simulink model "FowardDynamics_CDPR_20220518"  (R2020a)
settings: Solver=VariableStepAuto  StartTime=0.0  StopTime=12  FixedStep=0.01  RelTol=1e-3
undefined symbols (not defined in the file or in its folder): sigbuilder_block, X, Y, Z
libraries: sm_lib x197, nesl_utility x56, sm_cable_robot_lib x44, simulink x1
(part 2 of 8)

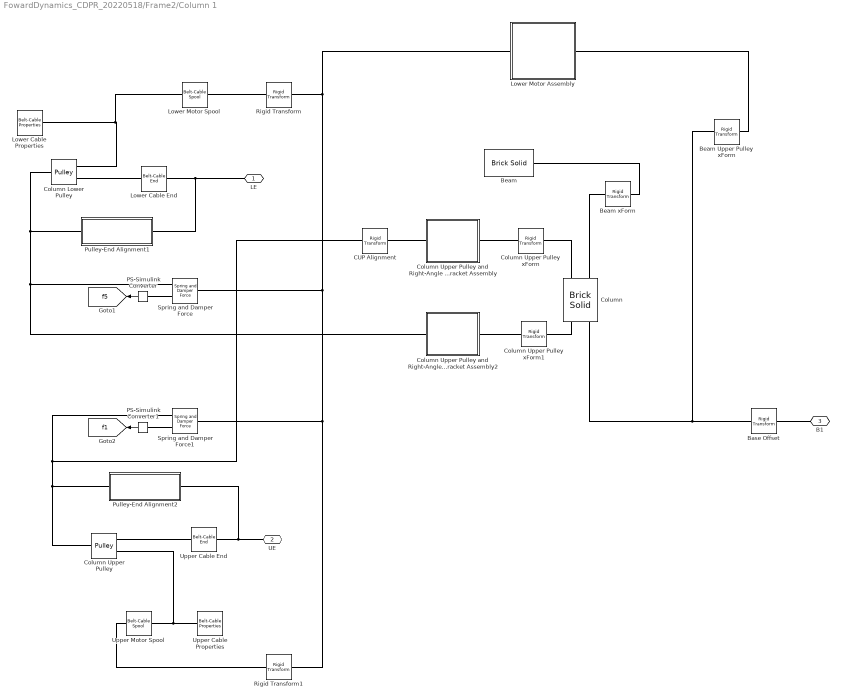
== system FowardDynamics_CDPR_20220518/Frame2/Column 1 ==
  Base Offset : sm_lib/Frames and Transforms/Rigid Transform  TranslationMethod=StandardAxis  TranslationStandardOffset=0  TranslationLengthUnit=m  TranslationStandardAxis=+X  TranslationCartesianOffset=[0 0 0]  TranslationROffset=0  TranslationROffsetUnits=m  TranslationZOffset=0  TranslationZOffsetUnits=m  TranslationThetaOffset=0  TranslationThetaOffsetUnits=deg  RotationMethod=None  RotationAngleUnits=deg  RotationStandardAxis=+Z  RotationAngle=0.0  RotationArbitraryAxis=[0 0 1]  FollAlignAxisA=+X  BaseAlignAxisA=+Y  FollAlignAxisB=+Y  BaseAlignAxisB=+Z  RotationSequenceAxes=FollowerAxes  RotationSequence=XYX  RotationSequenceAngles=[0 0 0]  RotationSequenceAnglesUnits=deg  RotationMatrix=[1 0 0; 0 1 0; 0 0 1]
  Beam : sm_lib/Body Elements/Brick Solid  GraphicAmbientColor=[0.15 0.15 0.15 1.0]  BasedOnType=Density  BrickDimensions=[0.1 2.1 0.1]  BrickDimensionUnits=m  CenterOfMass=[0 0 0]  CenterOfMassUnits=m  GraphicDiffuseColor=[0.4 0.4 0.4]  Density=7500  DensityUnits=kg/m^3  DoExposeReferenceFrame=off  GraphicEmissiveColor=[0.0 0.0 0.0 1.0]  ExportEntireGeometry=off  SerializedFrames=<Frames><Frame><Id>Frame3</Id><Value><Name>L</Name><Origin><Source>GeometricFeature</Source><FeatureName>-y surface</FeatureName></Origin><PrimaryAxis><DefinedDirection>+Z</DefinedDirection><Source>ReferenceFrame</Source><SourceDirection>+Z</SourceDirection><FeatureName></FeatureName></PrimaryAxis><SecondaryAxis><DefinedDirection>+X</DefinedDirection><Source>ReferenceFrame</Source><SourceDirection>+X</SourceDirection><FeatureName></FeatureName></SecondaryAxis></Value></Frame></Frames>  MarkerShape=Sphere  MarkerSize=10  GraphicType=FromGeometry  InertiaType=CalculateFromGeometry  Mass=1  MassUnits=kg  MomentsOfInertia=[1 1 1]  MomentsOfInertiaUnits=kg*m^2  GraphicOpacity=1.0  ProductsOfInertia=[0 0 0]  ProductsOfInertiaUnits=kg*m^2  GraphicShininess=75  GraphicSpecularColor=[0.5 0.5 0.5 1.0]  GraphicVisPropType=SimpleVisualProperties
  Beam Upper Pulley xForm : sm_lib/Frames and Transforms/Rigid Transform  TranslationMethod=Cartesian  TranslationStandardOffset=0.2  TranslationLengthUnit=m  TranslationStandardAxis=+X  TranslationCartesianOffset=[0.025 0.2 0]  TranslationROffset=0  TranslationROffsetUnits=m  TranslationZOffset=0  TranslationZOffsetUnits=m  TranslationThetaOffset=0  TranslationThetaOffsetUnits=deg  RotationMethod=RotationSequence  RotationAngleUnits=deg  RotationStandardAxis=+Y  RotationAngle=45  RotationArbitraryAxis=[0 0 1]  FollAlignAxisA=+X  BaseAlignAxisA=+Z  FollAlignAxisB=+Y  BaseAlignAxisB=-X  RotationSequenceAxes=FollowerAxes  RotationSequence=XYZ  RotationSequenceAngles=[90 45 0]  RotationSequenceAnglesUnits=deg  RotationMatrix=[1 0 0; 0 1 0; 0 0 1]
  Beam xForm : sm_lib/Frames and Transforms/Rigid Transform  TranslationMethod=Cartesian  TranslationStandardOffset=0  TranslationLengthUnit=m  TranslationStandardAxis=+X  TranslationCartesianOffset=[0 0 0.05]  TranslationROffset=0  TranslationROffsetUnits=m  TranslationZOffset=0  TranslationZOffsetUnits=m  TranslationThetaOffset=0  TranslationThetaOffsetUnits=deg  RotationMethod=None  RotationAngleUnits=deg  RotationStandardAxis=+Z  RotationAngle=0.0  RotationArbitraryAxis=[0 0 1]  FollAlignAxisA=+X  BaseAlignAxisA=+Y  FollAlignAxisB=+Y  BaseAlignAxisB=+Z  RotationSequenceAxes=FollowerAxes  RotationSequence=XYX  RotationSequenceAngles=[0 0 0]  RotationSequenceAnglesUnits=deg  RotationMatrix=[1 0 0; 0 1 0; 0 0 1]
  CUP Alignment : sm_lib/Frames and Transforms/Rigid Transform  TranslationMethod=None  TranslationStandardOffset=0  TranslationLengthUnit=m  TranslationStandardAxis=+Z  TranslationCartesianOffset=[0 0 0]  TranslationROffset=0  TranslationROffsetUnits=m  TranslationZOffset=0  TranslationZOffsetUnits=m  TranslationThetaOffset=0  TranslationThetaOffsetUnits=deg  RotationMethod=AlignedAxes  RotationAngleUnits=deg  RotationStandardAxis=+Z  RotationAngle=0.0  RotationArbitraryAxis=[0 0 1]  FollAlignAxisA=+Z  BaseAlignAxisA=-Z  FollAlignAxisB=+X  BaseAlignAxisB=+X  RotationSequenceAxes=FollowerAxes  RotationSequence=XYX  RotationSequenceAngles=[0 0 0]  RotationSequenceAnglesUnits=deg  RotationMatrix=[1 0 0; 0 1 0; 0 0 1]
  Column : sm_lib/Body Elements/Brick Solid  GraphicAmbientColor=[0.15 0.15 0.15 1.0]  BasedOnType=Density  BrickDimensions=[0.1 0.1 1.6]  BrickDimensionUnits=m  CenterOfMass=[0 0 0]  CenterOfMassUnits=m  GraphicDiffuseColor=[0.4 0.4 0.4]  Density=7900  DensityUnits=kg/m^3  DoExposeReferenceFrame=off  GraphicEmissiveColor=[0.0 0.0 0.0 1.0]  ExportEntireGeometry=off  SerializedFrames=<Frames><Frame><Id>Frame1</Id><Value><Name>LP</Name><Origin><Source>GeometricFeature</Source><FeatureName>+x surface</FeatureName></Origin><PrimaryAxis><DefinedDirection>+Z</DefinedDirection><Source>ReferenceFrame</Source><SourceDirection>+Z</SourceDirection><FeatureName></FeatureName></PrimaryAxis><SecondaryAxis><DefinedDirection>+X</DefinedDirection><Source>ReferenceFrame</Source><SourceDirection>-Y</SourceDirection><FeatureName></FeatureName></SecondaryAxis></Value></Frame><Frame><Id>Frame2</Id><Value><Name>UP</Name><Origin><Source>GeometricFeature</Source><FeatureName>+z +x curve</FeatureName></Origin><PrimaryAxis><DefinedDirection>+Z</DefinedDirection><Source>ReferenceFrame</Source><SourceDirection>+Z</SourceDirection><FeatureName></FeatureName></PrimaryAxis><SecondaryAxis><DefinedDirection>+X</DefinedDirection><Source>ReferenceFrame</Source><SourceDirection>-Y</SourceDirection><FeatureName></FeatureName></SecondaryAxis></Value></Frame><Frame><Id>Frame3</Id><Value><Name>B</Name><Origin><Source>GeometricFeature</Source><FeatureName>-x -y -z point</FeatureName></Origin><PrimaryAxis><DefinedDirection>+Z</DefinedDirection><Source>ReferenceFrame</Source><SourceDirection>+Z</SourceDirection><FeatureName></FeatureName></PrimaryAxis><SecondaryAxis><DefinedDirection>+X</DefinedDirection><Source>ReferenceFrame</Source><SourceDirection>+X</SourceDirection><FeatureName></FeatureName></SecondaryAxis></Value></Frame><Frame><Id>Frame4</Id><Value><Name>M1</Name><Origin><Source>GeometricFeature</Source><FeatureName>+z +x curve</FeatureName></Origin><PrimaryAxis><DefinedDirection>+Z</DefinedDirection><Source>ReferenceFrame</Source><SourceDirection>+Z</SourceDirection><FeatureName></FeatureName></PrimaryAxis><SecondaryAxis><DefinedDirection>+X</DefinedDirection><Source>ReferenceFrame</Source><SourceDirection>-Y</SourceDirection><FeatureName></FeatureName></SecondaryAxis></Value></Frame></Frames>  MarkerShape=Sphere  MarkerSize=10  GraphicType=FromGeometry  InertiaType=CalculateFromGeometry  Mass=1  MassUnits=kg  MomentsOfInertia=[1 1 1]  MomentsOfInertiaUnits=kg*m^2  GraphicOpacity=1.0  ProductsOfInertia=[0 0 0]  ProductsOfInertiaUnits=kg*m^2  GraphicShininess=75  GraphicSpecularColor=[0.5 0.5 0.5 1.0]  GraphicVisPropType=SimpleVisualProperties
  Column Lower Pulley : sm_lib/Belts and Cables/Pulley  PitchRadius=0.038  PitchRadiusUnits=m  InitialWrapAngleLowerBound=0.0  InitialWrapAngleLowerBoundUnits=deg  SenseWrapAngle=off  SensePulleyAngleA=off  SensePulleyAngleB=off  SenseFleetAngleA=off  SenseFleetAngleB=off
      settings: SourceProductBaseCode=MS
  Column Upper Pulley : sm_lib/Belts and Cables/Pulley  PitchRadius=0.038  PitchRadiusUnits=m  InitialWrapAngleLowerBound=0.0  InitialWrapAngleLowerBoundUnits=deg  SenseWrapAngle=off  SensePulleyAngleA=off  SensePulleyAngleB=off  SenseFleetAngleA=off  SenseFleetAngleB=off
      settings: SourceProductBaseCode=MS
  Column Upper Pulley xForm : sm_lib/Frames and Transforms/Rigid Transform  TranslationMethod=Cartesian  TranslationStandardOffset=0.2  TranslationLengthUnit=m  TranslationStandardAxis=-Z  TranslationCartesianOffset=[-0.035 0 -0.1]  TranslationROffset=0  TranslationROffsetUnits=m  TranslationZOffset=0  TranslationZOffsetUnits=m  TranslationThetaOffset=0  TranslationThetaOffsetUnits=deg  RotationMethod=AlignedAxes  RotationAngleUnits=deg  RotationStandardAxis=+Z  RotationAngle=0.0  RotationArbitraryAxis=[0 0 1]  FollAlignAxisA=+Z  BaseAlignAxisA=+Y  FollAlignAxisB=+X  BaseAlignAxisB=-X  RotationSequenceAxes=FollowerAxes  RotationSequence=XYX  RotationSequenceAngles=[0 0 0]  RotationSequenceAnglesUnits=deg  RotationMatrix=[1 0 0; 0 1 0; 0 0 1]
  Column Upper Pulley xForm1 : sm_lib/Frames and Transforms/Rigid Transform  TranslationMethod=Cartesian  TranslationStandardOffset=0.2  TranslationLengthUnit=m  TranslationStandardAxis=-Z  TranslationCartesianOffset=[-0.035 0 0.6]  TranslationROffset=0  TranslationROffsetUnits=m  TranslationZOffset=0  TranslationZOffsetUnits=m  TranslationThetaOffset=0  TranslationThetaOffsetUnits=deg  RotationMethod=AlignedAxes  RotationAngleUnits=deg  RotationStandardAxis=+Z  RotationAngle=0.0  RotationArbitraryAxis=[0 0 1]  FollAlignAxisA=+Z  BaseAlignAxisA=+Y  FollAlignAxisB=+X  BaseAlignAxisB=-X  RotationSequenceAxes=FollowerAxes  RotationSequence=XYX  RotationSequenceAngles=[0 0 0]  RotationSequenceAnglesUnits=deg  RotationMatrix=[1 0 0; 0 1 0; 0 0 1]
  Column Upper Pulley and Right-Angle Bracket Assembly : Subsystem  AncestorBlock=sm_cable_robot_lib/Pulley and Right-Angle Bracket Assembly  mask(Pulley and Right-Angle Bracket Assembly){baseBracketHeight=0.022, baseBracketWidth=0.022, baseBracketThickness=0.005, baseBracketOffset=0.024, baseBracketHoleOffset=0.012, baseBracketHoleRadius=0.005, rightBracketWidth=0.015, rightBracketHeight=0.06, rightBracketLegLength=0.04, rightBracketHoleOffset=0.05, pulleyRadius=0.04, pulleyThickness=0.01, pulleyHoleRadius=0.005, pulleyGrooveDepth=0.004, pulleyGrooveWidth=0.005, pulleyGrooveAngle=25, bracketRho=7800, pulleyRho=7800, pinRho=7800, bracketColor=[0.3 0.3 0.3], pulleyColor=[1.0 1.0 0.0], pulleyMarkerColor=[0.3 0.3 0.3], pinColor=[0.9 0.9 0.9]}
      mask prompts: baseBracketHeight "Height (m)"; baseBracketWidth "Width (m)"; baseBracketThickness "Thickness (m)"; baseBracketOffset "Offset (m)"; baseBracketHoleOffset "Hole Offset (m)"; baseBracketHoleRadius "Hole Radius (m)"; rightBracketWidth "Width (m)"; rightBracketHeight "Height (m)"; rightBracketLegLength "Leg Length (m)"; rightBracketHoleOffset "Hole Offset (m)"; pulleyRadius "Radius (m)"; pulleyThickness "Thickness (m)"; pulleyHoleRadius "Hole Radius (m)"; pulleyGrooveDepth "Groove Depth (m)"; pulleyGrooveWidth "Groove Width (m)"; pulleyGrooveAngle "Groove Angle (deg)"; bracketRho "Bracket Density (kg/m^3)"; pulleyRho "Pulley Density (kg/m^3)"; pinRho "Pin Density (kg/m^3)"; bracketColor "Bracket Color [r g b]"; pulleyColor "Pulley Color [r g b]"; pulleyMarkerColor "Pulley Marker Color [r g b]"; pinColor "Pin Color [r g b]"
      mask help:
      | This blocks models a pulley and right-angle bracket assembly. The pulley is connected to the right-angle bracket via a revolute joint. The pulley axis is aligned with the right-angle bracket hole axis. The right-angle bracket is connected to a pair of double brackets, with the right-angle bracket rigidly connected to one, and the other is connected to the first double bracket via a revolute joint.
      |
      | Port B corresponds to the base of the second double bracket. Port P corresponds to the reference frame of the pulley.
      mask init:
      | rightBracketOffset    = baseBracketWidth - baseBracketThickness;
      | follBracketOffset     = baseBracketOffset - 2 * baseBracketThickness;
      | follBracketHeight     = baseBracketHeight - baseBracketThickness;
      | follBracketHoleOffset = baseBracketHoleOffset - baseBracketThickness;
      | 
      | swivelPinLength       = baseBracketOffset  + baseBracketThickness;
      | pulleyPinLength       = rightBracketOffset + baseBracketThickness;
      mask DialogControl Tab1 Prompt: Base Bracket Dimensions
      mask DialogControl Tab2 Prompt: Right-Angle Bracket Dimensions
      mask DialogControl Tab3 Prompt: Pulley Dimensions
      mask DialogControl Tab4 Prompt: Material Properties
      mask Display: image(fullfile(matlabroot,'toolbox','physmod','sm','smdemos','cable_robot','images','sm_cable_robot_pulley_right_bracket_assembly.png'));
  Column Upper Pulley and Right-Angle Bracket Assembly2 : Subsystem  AncestorBlock=sm_cable_robot_lib/Pulley and Right-Angle Bracket Assembly  mask(Pulley and Right-Angle Bracket Assembly){baseBracketHeight=0.022, baseBracketWidth=0.022, baseBracketThickness=0.005, baseBracketOffset=0.024, baseBracketHoleOffset=0.012, baseBracketHoleRadius=0.005, rightBracketWidth=0.015, rightBracketHeight=0.06, rightBracketLegLength=0.04, rightBracketHoleOffset=0.05, pulleyRadius=0.04, pulleyThickness=0.01, pulleyHoleRadius=0.005, pulleyGrooveDepth=0.004, pulleyGrooveWidth=0.005, pulleyGrooveAngle=25, bracketRho=7800, pulleyRho=7800, pinRho=7800, bracketColor=[0.3 0.3 0.3], pulleyColor=[1.0 1.0 0.0], pulleyMarkerColor=[0.3 0.3 0.3], pinColor=[0.9 0.9 0.9]}
      mask prompts: baseBracketHeight "Height (m)"; baseBracketWidth "Width (m)"; baseBracketThickness "Thickness (m)"; baseBracketOffset "Offset (m)"; baseBracketHoleOffset "Hole Offset (m)"; baseBracketHoleRadius "Hole Radius (m)"; rightBracketWidth "Width (m)"; rightBracketHeight "Height (m)"; rightBracketLegLength "Leg Length (m)"; rightBracketHoleOffset "Hole Offset (m)"; pulleyRadius "Radius (m)"; pulleyThickness "Thickness (m)"; pulleyHoleRadius "Hole Radius (m)"; pulleyGrooveDepth "Groove Depth (m)"; pulleyGrooveWidth "Groove Width (m)"; pulleyGrooveAngle "Groove Angle (deg)"; bracketRho "Bracket Density (kg/m^3)"; pulleyRho "Pulley Density (kg/m^3)"; pinRho "Pin Density (kg/m^3)"; bracketColor "Bracket Color [r g b]"; pulleyColor "Pulley Color [r g b]"; pulleyMarkerColor "Pulley Marker Color [r g b]"; pinColor "Pin Color [r g b]"
      mask help:
      | This blocks models a pulley and right-angle bracket assembly. The pulley is connected to the right-angle bracket via a revolute joint. The pulley axis is aligned with the right-angle bracket hole axis. The right-angle bracket is connected to a pair of double brackets, with the right-angle bracket rigidly connected to one, and the other is connected to the first double bracket via a revolute joint.
      |
      | Port B corresponds to the base of the second double bracket. Port P corresponds to the reference frame of the pulley.
      mask init: same as FowardDynamics_CDPR_20220518/Frame2/Column 1/Column Upper Pulley and Right-Angle Bracket Assembly
      mask DialogControl Tab1 Prompt: Base Bracket Dimensions
      mask DialogControl Tab2 Prompt: Right-Angle Bracket Dimensions
      mask DialogControl Tab3 Prompt: Pulley Dimensions
      mask DialogControl Tab4 Prompt: Material Properties
      mask Display: image(fullfile(matlabroot,'toolbox','physmod','sm','smdemos','cable_robot','images','sm_cable_robot_pulley_right_bracket_assembly.png'));
  Lower Cable End : sm_lib/Belts and Cables/Belt-Cable End
      settings: SourceProductBaseCode=MS
  Lower Cable Properties : sm_lib/Belts and Cables/Belt-Cable Properties  DrumBeltCableAlignment=MonitoredPlanar  GraphicType=PitchLine  GraphicVisPropType=SimpleVisualProperties  GraphicDiffuseColor=[1.0 1.0 1.0]  GraphicSpecularColor=[0.5 0.5 0.5 1.0]  GraphicAmbientColor=[0.15 0.15 0.15 1.0]  GraphicEmissiveColor=[0.0 0.0 0.0 1.0]  GraphicShininess=75  GraphicOpacity=1.0
      settings: SourceProductBaseCode=MS
  Lower Motor Spool : sm_lib/Belts and Cables/Belt-Cable Spool  PitchRadius=0.018  PitchRadiusUnits=m  SenseSpoolAngleA=off  SenseFleetAngleA=off
      settings: SourceProductBaseCode=MS
  Lower Motor Assembly : Subsystem  AncestorBlock=sm_cable_robot_lib/Motor Assembly  mask{motorWidth=0.05, motorHeight=0.05, motorDepth=0.1, motorShaftRadius=0.005, motorShaftLength=0.15, spoolAlignment=Right-Hand, spoolRadius=0.02, spoolThickness=0.2, spoolGrooveDepth=0.004, spoolGrooveWidth=0.1, spoolGrooveAngle=25, motorHousingRho=7800, motorShaftRho=7800, spoolRho=7800, motorHousingColor=[0.2 0.6 1.0], motorFlangeColor=[0.7 0.7 0.7], motorShaftColor=[0.9 0.9 0.9], spoolColor=[0.7 0.7 0.7], spoolMarkerColor=[0.3 0.3 0.3]}
      mask prompts: motorWidth "Width (m)"; motorHeight "Height (m)"; motorDepth "Depth (m)"; motorShaftRadius "Shaft Radius (m)"; motorShaftLength "Shaft Length (m)"; spoolAlignment "Spool Alignment"; spoolRadius "Radius (m)"; spoolThickness "Thickness (m)"; spoolGrooveDepth "Groove Depth (m)"; spoolGrooveWidth "Groove Width (m)"; spoolGrooveAngle "Groove Angle (deg)"; motorHousingRho "Motor Housing Density (kg/m^3)"; motorShaftRho "Motor Shaft Density (kg/m^3)"; spoolRho "Spool Density (kg/m^3)"; motorHousingColor "Motor Housing Color [r g b]"; motorFlangeColor "Motor Flange Color [r g b]"; motorShaftColor "Motor Shaft Color [r g b]"; spoolColor "Spool Color [r g b]"; spoolMarkerColor "Spool Marker Color [r g b]"
      mask init:
      | blk = gcb;
      | 
      | if spoolAlignment == 1
      |   set_param([blk '/Spool Alignment'],'BaseAlignAxisA','+Z');
      | else
      |   set_param([blk '/Spool Alignment'],'BaseAlignAxisA','-Z');
      | end
      mask TypeOptions spoolAlignment: Right-Hand | Left-Hand
      mask DialogControl Tab1 Prompt: Motor Dimensions
      mask DialogControl Tab2 Prompt: Spool Dimensions
      mask DialogControl Tab3 Prompt: Material Properties
      mask Display: image(fullfile(matlabroot,'toolbox','physmod','sm','smdemos','cable_robot','images','sm_cable_robot_motor_assembly.png'));
  PS-Simulink Converter : nesl_utility/PS-Simulink Converter  PhysicalDomain=network_engine_domain  SubClassName=ps_output  LeftPortType=input  RightPortType=output  PseudoPeriodic=off  Frequencies=[]  Unit=inherit  AffineConversion=off
  PS-Simulink Converter1 : nesl_utility/PS-Simulink Converter  PhysicalDomain=network_engine_domain  SubClassName=ps_output  LeftPortType=input  RightPortType=output  PseudoPeriodic=off  Frequencies=[]  Unit=inherit  AffineConversion=off
  Pulley-End Alignment1 : Subsystem  AncestorBlock=sm_cable_robot_lib/Pulley-End Alignment  mask(Pulley-End Alignment){majorRadius=0.003, minorRadius=0.001, rho=7800, color=[0.3 0.3 0.3]}
      mask prompts: majorRadius "Ring Major Radius (m)"; minorRadius "Ring Minor Radius (m)"; rho "Ring Density (kg/m^3)"; color "Ring Color [r g b]"
      mask help:
      | This block models the enforced alignment between the belt-cable end attached to the mover and the corresponding column pulley. The block maintains the alignment between the belt-cable and the column pulley such that the belt-cable is always in the x-y plane of the column pulley.
      |
      | Port P corresponds to the pulley reference frame. Port E corresponds to the belt-cable end reference frame.
      mask init:
      | theta = linspace(0, 2 * pi, 20);
      | 
      | crossSection = [minorRadius * cos(theta) + majorRadius;...
      |                 minorRadius * sin(theta)]';
      mask DialogControl Tab1 Prompt: Dimensions
      mask DialogControl Tab2 Prompt: Material Properties
      mask Display: image(fullfile(matlabroot,'toolbox','physmod','sm','smdemos','cable_robot','images','sm_cable_robot_pulley_end_alignment.png'));
  Pulley-End Alignment2 : Subsystem  AncestorBlock=sm_cable_robot_lib/Pulley-End Alignment  mask(Pulley-End Alignment){majorRadius=0.003, minorRadius=0.001, rho=7800, color=[0.3 0.3 0.3]}
      mask prompts: majorRadius "Ring Major Radius (m)"; minorRadius "Ring Minor Radius (m)"; rho "Ring Density (kg/m^3)"; color "Ring Color [r g b]"
      mask help:
      | This block models the enforced alignment between the belt-cable end attached to the mover and the corresponding column pulley. The block maintains the alignment between the belt-cable and the column pulley such that the belt-cable is always in the x-y plane of the column pulley.
      |
      | Port P corresponds to the pulley reference frame. Port E corresponds to the belt-cable end reference frame.
      mask init:
      | theta = linspace(0, 2 * pi, 20);
      | 
      | crossSection = [minorRadius * cos(theta) + majorRadius;...
      |                 minorRadius * sin(theta)]';
      mask DialogControl Tab1 Prompt: Dimensions
      mask DialogControl Tab2 Prompt: Material Properties
      mask Display: image(fullfile(matlabroot,'toolbox','physmod','sm','smdemos','cable_robot','images','sm_cable_robot_pulley_end_alignment.png'));
  Rigid Transform : sm_lib/Frames and Transforms/Rigid Transform  TranslationMethod=StandardAxis  TranslationStandardOffset=0.03535  TranslationLengthUnit=m  TranslationStandardAxis=+Z  TranslationCartesianOffset=[0 0 0]  TranslationROffset=0  TranslationROffsetUnits=m  TranslationZOffset=0  TranslationZOffsetUnits=m  TranslationThetaOffset=0  TranslationThetaOffsetUnits=deg  RotationMethod=None  RotationAngleUnits=deg  RotationStandardAxis=+Z  RotationAngle=0.0  RotationArbitraryAxis=[0 0 1]  FollAlignAxisA=+X  BaseAlignAxisA=+Y  FollAlignAxisB=+Y  BaseAlignAxisB=+Z  RotationSequenceAxes=FollowerAxes  RotationSequence=XYX  RotationSequenceAngles=[0 0 0]  RotationSequenceAnglesUnits=deg  RotationMatrix=[1 0 0; 0 1 0; 0 0 1]
  Rigid Transform1 : sm_lib/Frames and Transforms/Rigid Transform  TranslationMethod=StandardAxis  TranslationStandardOffset=0.03535  TranslationLengthUnit=m  TranslationStandardAxis=-Z  TranslationCartesianOffset=[0 0 0]  TranslationROffset=0  TranslationROffsetUnits=m  TranslationZOffset=0  TranslationZOffsetUnits=m  TranslationThetaOffset=0  TranslationThetaOffsetUnits=deg  RotationMethod=None  RotationAngleUnits=deg  RotationStandardAxis=+Z  RotationAngle=0.0  RotationArbitraryAxis=[0 0 1]  FollAlignAxisA=+X  BaseAlignAxisA=+Y  FollAlignAxisB=+Y  BaseAlignAxisB=+Z  RotationSequenceAxes=FollowerAxes  RotationSequence=XYX  RotationSequenceAngles=[0 0 0]  RotationSequenceAnglesUnits=deg  RotationMatrix=[1 0 0; 0 1 0; 0 0 1]
  Spring and Damper Force : sm_lib/Forces and Torques/Spring and Damper Force  NaturalLength=2  NaturalLengthUnits=m  SpringStiffness=115  SpringStiffnessUnits=N/m  DampingCoefficient=0.2  DampingCoefficientUnits=N/(m/s)  SenseForce=on
  Spring and Damper Force1 : sm_lib/Forces and Torques/Spring and Damper Force  NaturalLength=2  NaturalLengthUnits=m  SpringStiffness=150  SpringStiffnessUnits=N/m  DampingCoefficient=0.2  DampingCoefficientUnits=N/(m/s)  SenseForce=on
  Upper Cable End : sm_lib/Belts and Cables/Belt-Cable End
      settings: SourceProductBaseCode=MS
  Upper Cable Properties : sm_lib/Belts and Cables/Belt-Cable Properties  DrumBeltCableAlignment=MonitoredPlanar  GraphicType=PitchLine  GraphicVisPropType=SimpleVisualProperties  GraphicDiffuseColor=[1.0 1.0 1.0]  GraphicSpecularColor=[0.5 0.5 0.5 1.0]  GraphicAmbientColor=[0.15 0.15 0.15 1.0]  GraphicEmissiveColor=[0.0 0.0 0.0 1.0]  GraphicShininess=75  GraphicOpacity=1.0
      settings: SourceProductBaseCode=MS
  Upper Motor Spool : sm_lib/Belts and Cables/Belt-Cable Spool  PitchRadius=0.018  PitchRadiusUnits=m  SenseSpoolAngleA=off  SenseFleetAngleA=off
      settings: SourceProductBaseCode=MS
  LE : PMIOPort  Side=Left
  UE : PMIOPort  Port=2  Side=Left
  B1 : PMIOPort  Port=3  Side=Right
  tag scope: f1=global, f5=global
  wires:
  PS-Simulink Converter/1 -> [f5]
  PS-Simulink Converter1/1 -> [f1]
  connections:
  Pulley-End Alignment2/RConn1 -- Upper Cable End/LConn1 -- UE/RConn1
  Pulley-End Alignment1/RConn1 -- Lower Cable End/LConn1 -- LE/RConn1
  Pulley-End Alignment2/LConn1 -- Spring and Damper Force1/RConn1 -- CUP Alignment/RConn1 -- Column Upper Pulley/LConn1
  Column Lower Pulley/RConn2 -- Lower Cable End/RConn1
  B1/RConn1 -- Base Offset/RConn1
  Column Upper Pulley xForm/LConn1 -- Column/RConn1
  Column Upper Pulley xForm1/LConn1 -- Column/LConn1
  Column/LConn2 -- Base Offset/LConn1 -- Beam Upper Pulley xForm/LConn1
  Lower Motor Assembly/LConn1 -- Beam Upper Pulley xForm/RConn1
  Beam xForm/LConn1 -- Column/RConn2
  Beam/LConn1 -- Beam xForm/RConn1
  Upper Motor Spool/RConn1 -- Column Upper Pulley/RConn2 -- Upper Cable Properties/LConn1
  Lower Cable Properties/LConn1 -- Lower Motor Spool/RConn1 -- Column Lower Pulley/RConn1
  Rigid Transform/LConn1 -- Spring and Damper Force1/LConn1 -- Rigid Transform1/LConn1 -- Spring and Damper Force/LConn1 -- Lower Motor Assembly/RConn1
  Column Upper Pulley/RConn1 -- Upper Cable End/RConn1
  Rigid Transform/RConn1 -- Lower Motor Spool/LConn1
  Rigid Transform1/RConn1 -- Upper Motor Spool/LConn1
  Column Lower Pulley/LConn1 -- Column Upper Pulley and Right-Angle Bracket Assembly2/RConn1 -- Spring and Damper Force/RConn1 -- Pulley-End Alignment1/LConn1
  Column Upper Pulley and Right-Angle Bracket Assembly/LConn1 -- Column Upper Pulley xForm/RConn1
  Column Upper Pulley xForm1/RConn1 -- Column Upper Pulley and Right-Angle Bracket Assembly2/LConn1
  CUP Alignment/LConn1 -- Column Upper Pulley and Right-Angle Bracket Assembly/RConn1
  PS-Simulink Converter/LConn1 -- Spring and Damper Force/RConn2
  PS-Simulink Converter1/LConn1 -- Spring and Damper Force1/RConn2

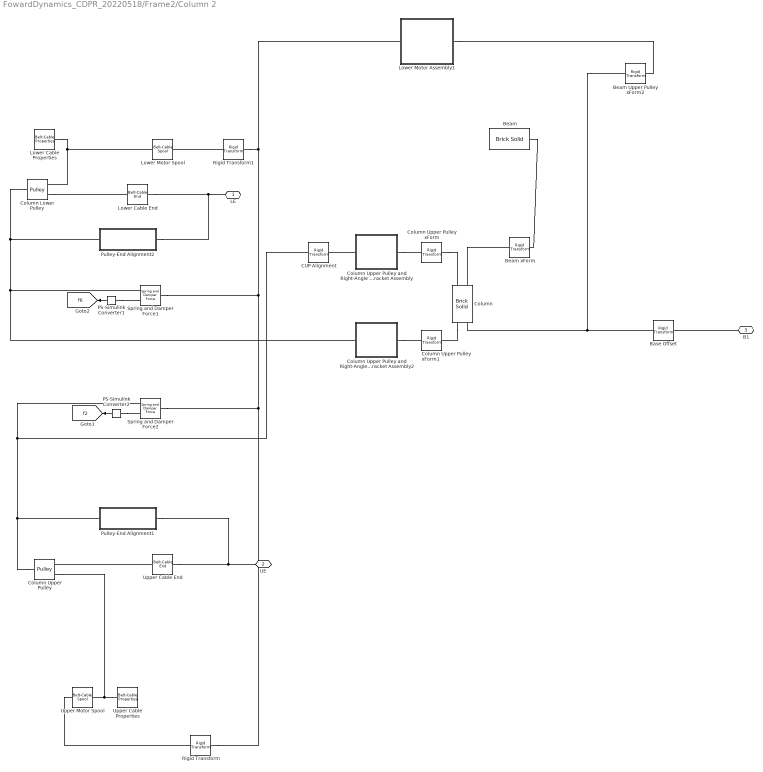
== system FowardDynamics_CDPR_20220518/Frame2/Column 2 ==
  Base Offset : sm_lib/Frames and Transforms/Rigid Transform  TranslationMethod=StandardAxis  TranslationStandardOffset=0  TranslationLengthUnit=m  TranslationStandardAxis=+X  TranslationCartesianOffset=[0 0 0]  TranslationROffset=0  TranslationROffsetUnits=m  TranslationZOffset=0  TranslationZOffsetUnits=m  TranslationThetaOffset=0  TranslationThetaOffsetUnits=deg  RotationMethod=None  RotationAngleUnits=deg  RotationStandardAxis=+Z  RotationAngle=0.0  RotationArbitraryAxis=[0 0 1]  FollAlignAxisA=+X  BaseAlignAxisA=+Y  FollAlignAxisB=+Y  BaseAlignAxisB=+Z  RotationSequenceAxes=FollowerAxes  RotationSequence=XYX  RotationSequenceAngles=[0 0 0]  RotationSequenceAnglesUnits=deg  RotationMatrix=[1 0 0; 0 1 0; 0 0 1]
  Beam : sm_lib/Body Elements/Brick Solid  GraphicAmbientColor=[0.15 0.15 0.15 1.0]  BasedOnType=Density  BrickDimensions=[0.1 2.9 0.1]  BrickDimensionUnits=m  CenterOfMass=[0 0 0]  CenterOfMassUnits=m  GraphicDiffuseColor=[0.4 0.4 0.4]  Density=7500  DensityUnits=kg/m^3  DoExposeReferenceFrame=off  GraphicEmissiveColor=[0.0 0.0 0.0 1.0]  ExportEntireGeometry=off  SerializedFrames=<Frames><Frame><Id>Frame3</Id><Value><Name>L</Name><Origin><Source>GeometricFeature</Source><FeatureName>-y surface</FeatureName></Origin><PrimaryAxis><DefinedDirection>+Z</DefinedDirection><Source>ReferenceFrame</Source><SourceDirection>+Z</SourceDirection><FeatureName></FeatureName></PrimaryAxis><SecondaryAxis><DefinedDirection>+X</DefinedDirection><Source>ReferenceFrame</Source><SourceDirection>+X</SourceDirection><FeatureName></FeatureName></SecondaryAxis></Value></Frame></Frames>  MarkerShape=Sphere  MarkerSize=10  GraphicType=FromGeometry  InertiaType=CalculateFromGeometry  Mass=1  MassUnits=kg  MomentsOfInertia=[1 1 1]  MomentsOfInertiaUnits=kg*m^2  GraphicOpacity=1.0  ProductsOfInertia=[0 0 0]  ProductsOfInertiaUnits=kg*m^2  GraphicShininess=75  GraphicSpecularColor=[0.5 0.5 0.5 1.0]  GraphicVisPropType=SimpleVisualProperties
  Beam Upper Pulley xForm2 : sm_lib/Frames and Transforms/Rigid Transform  TranslationMethod=Cartesian  TranslationStandardOffset=0.2  TranslationLengthUnit=m  TranslationStandardAxis=+X  TranslationCartesianOffset=[-0.025,0.2 0]  TranslationROffset=0  TranslationROffsetUnits=m  TranslationZOffset=0  TranslationZOffsetUnits=m  TranslationThetaOffset=0  TranslationThetaOffsetUnits=deg  RotationMethod=RotationSequence  RotationAngleUnits=deg  RotationStandardAxis=+Y  RotationAngle=45  RotationArbitraryAxis=[0 0 1]  FollAlignAxisA=+X  BaseAlignAxisA=+Z  FollAlignAxisB=+Y  BaseAlignAxisB=-X  RotationSequenceAxes=FollowerAxes  RotationSequence=XYZ  RotationSequenceAngles=[90 -45 0]  RotationSequenceAnglesUnits=deg  RotationMatrix=[1 0 0; 0 1 0; 0 0 1]
  Beam xForm : sm_lib/Frames and Transforms/Rigid Transform  TranslationMethod=Cartesian  TranslationStandardOffset=0  TranslationLengthUnit=m  TranslationStandardAxis=+X  TranslationCartesianOffset=[0 0 0.05]  TranslationROffset=0  TranslationROffsetUnits=m  TranslationZOffset=0  TranslationZOffsetUnits=m  TranslationThetaOffset=0  TranslationThetaOffsetUnits=deg  RotationMethod=None  RotationAngleUnits=deg  RotationStandardAxis=+Z  RotationAngle=0.0  RotationArbitraryAxis=[0 0 1]  FollAlignAxisA=+X  BaseAlignAxisA=+Y  FollAlignAxisB=+Y  BaseAlignAxisB=+Z  RotationSequenceAxes=FollowerAxes  RotationSequence=XYX  RotationSequenceAngles=[0 0 0]  RotationSequenceAnglesUnits=deg  RotationMatrix=[1 0 0; 0 1 0; 0 0 1]
  CUP Alignment : sm_lib/Frames and Transforms/Rigid Transform  TranslationMethod=None  TranslationStandardOffset=0  TranslationLengthUnit=m  TranslationStandardAxis=+Z  TranslationCartesianOffset=[0 0 0]  TranslationROffset=0  TranslationROffsetUnits=m  TranslationZOffset=0  TranslationZOffsetUnits=m  TranslationThetaOffset=0  TranslationThetaOffsetUnits=deg  RotationMethod=AlignedAxes  RotationAngleUnits=deg  RotationStandardAxis=+Z  RotationAngle=0.0  RotationArbitraryAxis=[0 0 1]  FollAlignAxisA=+Z  BaseAlignAxisA=-Z  FollAlignAxisB=+X  BaseAlignAxisB=+X  RotationSequenceAxes=FollowerAxes  RotationSequence=XYX  RotationSequenceAngles=[0 0 0]  RotationSequenceAnglesUnits=deg  RotationMatrix=[1 0 0; 0 1 0; 0 0 1]
  Column : sm_lib/Body Elements/Brick Solid  GraphicAmbientColor=[0.15 0.15 0.15 1.0]  BasedOnType=Density  BrickDimensions=[0.1 0.1 1.6]  BrickDimensionUnits=m  CenterOfMass=[0 0 0]  CenterOfMassUnits=m  GraphicDiffuseColor=[0.4 0.4 0.4]  Density=7900  DensityUnits=kg/m^3  DoExposeReferenceFrame=off  GraphicEmissiveColor=[0.0 0.0 0.0 1.0]  ExportEntireGeometry=off  SerializedFrames=<Frames><Frame><Id>Frame1</Id><Value><Name>LP</Name><Origin><Source>GeometricFeature</Source><FeatureName>+y surface</FeatureName></Origin><PrimaryAxis><DefinedDirection>+Z</DefinedDirection><Source>ReferenceFrame</Source><SourceDirection>+Z</SourceDirection><FeatureName></FeatureName></PrimaryAxis><SecondaryAxis><DefinedDirection>+X</DefinedDirection><Source>ReferenceFrame</Source><SourceDirection>+X</SourceDirection><FeatureName></FeatureName></SecondaryAxis></Value></Frame><Frame><Id>Frame2</Id><Value><Name>UP</Name><Origin><Source>GeometricFeature</Source><FeatureName>+y +z curve</FeatureName></Origin><PrimaryAxis><DefinedDirection>+Z</DefinedDirection><Source>ReferenceFrame</Source><SourceDirection>+Z</SourceDirection><FeatureName></FeatureName></PrimaryAxis><SecondaryAxis><DefinedDirection>+X</DefinedDirection><Source>ReferenceFrame</Source><SourceDirection>+X</SourceDirection><FeatureName></FeatureName></SecondaryAxis></Value></Frame><Frame><Id>Frame3</Id><Value><Name>B</Name><Origin><Source>GeometricFeature</Source><FeatureName>-x -y -z point</FeatureName></Origin><PrimaryAxis><DefinedDirection>+Z</DefinedDirection><Source>ReferenceFrame</Source><SourceDirection>+Z</SourceDirection><FeatureName></FeatureName></PrimaryAxis><SecondaryAxis><DefinedDirection>+X</DefinedDirection><Source>ReferenceFrame</Source><SourceDirection>-Y</SourceDirection><FeatureName></FeatureName></SecondaryAxis></Value></Frame><Frame><Id>Frame4</Id><Value><Name>M</Name><Origin><Source>GeometricFeature</Source><FeatureName>+z +x curve</FeatureName></Origin><PrimaryAxis><DefinedDirection>+Z</DefinedDirection><Source>ReferenceFrame</Source><SourceDirection>+Z</SourceDirection><FeatureName></FeatureName></PrimaryAxis><SecondaryAxis><DefinedDirection>+X</DefinedDirection><Source>ReferenceFrame</Source><SourceDirection>-Y</SourceDirection><FeatureName></FeatureName></SecondaryAxis></Value></Frame></Frames>  MarkerShape=Sphere  MarkerSize=10  GraphicType=FromGeometry  InertiaType=CalculateFromGeometry  Mass=1  MassUnits=kg  MomentsOfInertia=[1 1 1]  MomentsOfInertiaUnits=kg*m^2  GraphicOpacity=1.0  ProductsOfInertia=[0 0 0]  ProductsOfInertiaUnits=kg*m^2  GraphicShininess=75  GraphicSpecularColor=[0.5 0.5 0.5 1.0]  GraphicVisPropType=SimpleVisualProperties
  Column Lower Pulley : sm_lib/Belts and Cables/Pulley  PitchRadius=0.038  PitchRadiusUnits=m  InitialWrapAngleLowerBound=0.0  InitialWrapAngleLowerBoundUnits=deg  SenseWrapAngle=off  SensePulleyAngleA=off  SensePulleyAngleB=off  SenseFleetAngleA=off  SenseFleetAngleB=off
      settings: SourceProductBaseCode=MS
  Column Upper Pulley : sm_lib/Belts and Cables/Pulley  PitchRadius=0.038  PitchRadiusUnits=m  InitialWrapAngleLowerBound=0.0  InitialWrapAngleLowerBoundUnits=deg  SenseWrapAngle=off  SensePulleyAngleA=off  SensePulleyAngleB=off  SenseFleetAngleA=off  SenseFleetAngleB=off
      settings: SourceProductBaseCode=MS
  Column Upper Pulley xForm : sm_lib/Frames and Transforms/Rigid Transform  TranslationMethod=Cartesian  TranslationStandardOffset=0.2  TranslationLengthUnit=m  TranslationStandardAxis=-Z  TranslationCartesianOffset=[0.035 0 -0.1]  TranslationROffset=0  TranslationROffsetUnits=m  TranslationZOffset=0  TranslationZOffsetUnits=m  TranslationThetaOffset=0  TranslationThetaOffsetUnits=deg  RotationMethod=AlignedAxes  RotationAngleUnits=deg  RotationStandardAxis=+Z  RotationAngle=0.0  RotationArbitraryAxis=[0 0 1]  FollAlignAxisA=+Z  BaseAlignAxisA=+Y  FollAlignAxisB=+X  BaseAlignAxisB=-X  RotationSequenceAxes=FollowerAxes  RotationSequence=XYX  RotationSequenceAngles=[0 0 0]  RotationSequenceAnglesUnits=deg  RotationMatrix=[1 0 0; 0 1 0; 0 0 1]
  Column Upper Pulley xForm1 : sm_lib/Frames and Transforms/Rigid Transform  TranslationMethod=Cartesian  TranslationStandardOffset=0.2  TranslationLengthUnit=m  TranslationStandardAxis=-Z  TranslationCartesianOffset=[0.035 0 0.6]  TranslationROffset=0  TranslationROffsetUnits=m  TranslationZOffset=0  TranslationZOffsetUnits=m  TranslationThetaOffset=0  TranslationThetaOffsetUnits=deg  RotationMethod=AlignedAxes  RotationAngleUnits=deg  RotationStandardAxis=+Z  RotationAngle=0.0  RotationArbitraryAxis=[0 0 1]  FollAlignAxisA=+Z  BaseAlignAxisA=+Y  FollAlignAxisB=+X  BaseAlignAxisB=-X  RotationSequenceAxes=FollowerAxes  RotationSequence=XYX  RotationSequenceAngles=[0 0 0]  RotationSequenceAnglesUnits=deg  RotationMatrix=[1 0 0; 0 1 0; 0 0 1]
  Column Upper Pulley and Right-Angle Bracket Assembly : Subsystem  AncestorBlock=sm_cable_robot_lib/Pulley and Right-Angle Bracket Assembly  mask(Pulley and Right-Angle Bracket Assembly){baseBracketHeight=0.022, baseBracketWidth=0.022, baseBracketThickness=0.005, baseBracketOffset=0.024, baseBracketHoleOffset=0.012, baseBracketHoleRadius=0.005, rightBracketWidth=0.015, rightBracketHeight=0.06, rightBracketLegLength=0.04, rightBracketHoleOffset=0.05, pulleyRadius=0.04, pulleyThickness=0.01, pulleyHoleRadius=0.005, pulleyGrooveDepth=0.004, pulleyGrooveWidth=0.005, pulleyGrooveAngle=25, bracketRho=7800, pulleyRho=7800, pinRho=7800, bracketColor=[0.3 0.3 0.3], pulleyColor=[1.0 1.0 0.0], pulleyMarkerColor=[0.3 0.3 0.3], pinColor=[0.9 0.9 0.9]}
      mask prompts: baseBracketHeight "Height (m)"; baseBracketWidth "Width (m)"; baseBracketThickness "Thickness (m)"; baseBracketOffset "Offset (m)"; baseBracketHoleOffset "Hole Offset (m)"; baseBracketHoleRadius "Hole Radius (m)"; rightBracketWidth "Width (m)"; rightBracketHeight "Height (m)"; rightBracketLegLength "Leg Length (m)"; rightBracketHoleOffset "Hole Offset (m)"; pulleyRadius "Radius (m)"; pulleyThickness "Thickness (m)"; pulleyHoleRadius "Hole Radius (m)"; pulleyGrooveDepth "Groove Depth (m)"; pulleyGrooveWidth "Groove Width (m)"; pulleyGrooveAngle "Groove Angle (deg)"; bracketRho "Bracket Density (kg/m^3)"; pulleyRho "Pulley Density (kg/m^3)"; pinRho "Pin Density (kg/m^3)"; bracketColor "Bracket Color [r g b]"; pulleyColor "Pulley Color [r g b]"; pulleyMarkerColor "Pulley Marker Color [r g b]"; pinColor "Pin Color [r g b]"
      mask help:
      | This blocks models a pulley and right-angle bracket assembly. The pulley is connected to the right-angle bracket via a revolute joint. The pulley axis is aligned with the right-angle bracket hole axis. The right-angle bracket is connected to a pair of double brackets, with the right-angle bracket rigidly connected to one, and the other is connected to the first double bracket via a revolute joint.
      |
      | Port B corresponds to the base of the second double bracket. Port P corresponds to the reference frame of the pulley.
      mask init: same as FowardDynamics_CDPR_20220518/Frame2/Column 1/Column Upper Pulley and Right-Angle Bracket Assembly
      mask DialogControl Tab1 Prompt: Base Bracket Dimensions
      mask DialogControl Tab2 Prompt: Right-Angle Bracket Dimensions
      mask DialogControl Tab3 Prompt: Pulley Dimensions
      mask DialogControl Tab4 Prompt: Material Properties
      mask Display: image(fullfile(matlabroot,'toolbox','physmod','sm','smdemos','cable_robot','images','sm_cable_robot_pulley_right_bracket_assembly.png'));
  Column Upper Pulley and Right-Angle Bracket Assembly2 : Subsystem  AncestorBlock=sm_cable_robot_lib/Pulley and Right-Angle Bracket Assembly  mask(Pulley and Right-Angle Bracket Assembly){baseBracketHeight=0.022, baseBracketWidth=0.022, baseBracketThickness=0.005, baseBracketOffset=0.024, baseBracketHoleOffset=0.012, baseBracketHoleRadius=0.005, rightBracketWidth=0.015, rightBracketHeight=0.06, rightBracketLegLength=0.04, rightBracketHoleOffset=0.05, pulleyRadius=0.04, pulleyThickness=0.01, pulleyHoleRadius=0.005, pulleyGrooveDepth=0.004, pulleyGrooveWidth=0.005, pulleyGrooveAngle=25, bracketRho=7800, pulleyRho=7800, pinRho=7800, bracketColor=[0.3 0.3 0.3], pulleyColor=[1.0 1.0 0.0], pulleyMarkerColor=[0.3 0.3 0.3], pinColor=[0.9 0.9 0.9]}
      mask prompts: baseBracketHeight "Height (m)"; baseBracketWidth "Width (m)"; baseBracketThickness "Thickness (m)"; baseBracketOffset "Offset (m)"; baseBracketHoleOffset "Hole Offset (m)"; baseBracketHoleRadius "Hole Radius (m)"; rightBracketWidth "Width (m)"; rightBracketHeight "Height (m)"; rightBracketLegLength "Leg Length (m)"; rightBracketHoleOffset "Hole Offset (m)"; pulleyRadius "Radius (m)"; pulleyThickness "Thickness (m)"; pulleyHoleRadius "Hole Radius (m)"; pulleyGrooveDepth "Groove Depth (m)"; pulleyGrooveWidth "Groove Width (m)"; pulleyGrooveAngle "Groove Angle (deg)"; bracketRho "Bracket Density (kg/m^3)"; pulleyRho "Pulley Density (kg/m^3)"; pinRho "Pin Density (kg/m^3)"; bracketColor "Bracket Color [r g b]"; pulleyColor "Pulley Color [r g b]"; pulleyMarkerColor "Pulley Marker Color [r g b]"; pinColor "Pin Color [r g b]"
      mask help:
      | This blocks models a pulley and right-angle bracket assembly. The pulley is connected to the right-angle bracket via a revolute joint. The pulley axis is aligned with the right-angle bracket hole axis. The right-angle bracket is connected to a pair of double brackets, with the right-angle bracket rigidly connected to one, and the other is connected to the first double bracket via a revolute joint.
      |
      | Port B corresponds to the base of the second double bracket. Port P corresponds to the reference frame of the pulley.
      mask init: same as FowardDynamics_CDPR_20220518/Frame2/Column 1/Column Upper Pulley and Right-Angle Bracket Assembly
      mask DialogControl Tab1 Prompt: Base Bracket Dimensions
      mask DialogControl Tab2 Prompt: Right-Angle Bracket Dimensions
      mask DialogControl Tab3 Prompt: Pulley Dimensions
      mask DialogControl Tab4 Prompt: Material Properties
      mask Display: image(fullfile(matlabroot,'toolbox','physmod','sm','smdemos','cable_robot','images','sm_cable_robot_pulley_right_bracket_assembly.png'));
  Lower Cable End : sm_lib/Belts and Cables/Belt-Cable End
      settings: SourceProductBaseCode=MS
  Lower Cable Properties : sm_lib/Belts and Cables/Belt-Cable Properties  DrumBeltCableAlignment=MonitoredPlanar  GraphicType=PitchLine  GraphicVisPropType=SimpleVisualProperties  GraphicDiffuseColor=[1.0 1.0 1.0]  GraphicSpecularColor=[0.5 0.5 0.5 1.0]  GraphicAmbientColor=[0.15 0.15 0.15 1.0]  GraphicEmissiveColor=[0.0 0.0 0.0 1.0]  GraphicShininess=75  GraphicOpacity=1.0
      settings: SourceProductBaseCode=MS
  Lower Motor Spool : sm_lib/Belts and Cables/Belt-Cable Spool  PitchRadius=0.018  PitchRadiusUnits=m  SenseSpoolAngleA=off  SenseFleetAngleA=off
      settings: SourceProductBaseCode=MS
  Lower Motor Assembly1 : Subsystem  AncestorBlock=sm_cable_robot_lib/Motor Assembly  mask{motorWidth=0.05, motorHeight=0.05, motorDepth=0.1, motorShaftRadius=0.005, motorShaftLength=0.15, spoolAlignment=Left-Hand, spoolRadius=0.02, spoolThickness=0.2, spoolGrooveDepth=0.004, spoolGrooveWidth=0.1, spoolGrooveAngle=25, motorHousingRho=7800, motorShaftRho=7800, spoolRho=7800, motorHousingColor=[0.2 0.6 1.0], motorFlangeColor=[0.7 0.7 0.7], motorShaftColor=[0.9 0.9 0.9], spoolColor=[0.7 0.7 0.7], spoolMarkerColor=[0.3 0.3 0.3]}
      mask prompts: motorWidth "Width (m)"; motorHeight "Height (m)"; motorDepth "Depth (m)"; motorShaftRadius "Shaft Radius (m)"; motorShaftLength "Shaft Length (m)"; spoolAlignment "Spool Alignment"; spoolRadius "Radius (m)"; spoolThickness "Thickness (m)"; spoolGrooveDepth "Groove Depth (m)"; spoolGrooveWidth "Groove Width (m)"; spoolGrooveAngle "Groove Angle (deg)"; motorHousingRho "Motor Housing Density (kg/m^3)"; motorShaftRho "Motor Shaft Density (kg/m^3)"; spoolRho "Spool Density (kg/m^3)"; motorHousingColor "Motor Housing Color [r g b]"; motorFlangeColor "Motor Flange Color [r g b]"; motorShaftColor "Motor Shaft Color [r g b]"; spoolColor "Spool Color [r g b]"; spoolMarkerColor "Spool Marker Color [r g b]"
      mask init:
      | blk = gcb;
      | 
      | if spoolAlignment == 1
      |   set_param([blk '/Spool Alignment'],'BaseAlignAxisA','+Z');
      | else
      |   set_param([blk '/Spool Alignment'],'BaseAlignAxisA','-Z');
      | end
      mask TypeOptions spoolAlignment: Right-Hand | Left-Hand
      mask DialogControl Tab1 Prompt: Motor Dimensions
      mask DialogControl Tab2 Prompt: Spool Dimensions
      mask DialogControl Tab3 Prompt: Material Properties
      mask Display: image(fullfile(matlabroot,'toolbox','physmod','sm','smdemos','cable_robot','images','sm_cable_robot_motor_assembly.png'));
  PS-Simulink Converter1 : nesl_utility/PS-Simulink Converter  PhysicalDomain=network_engine_domain  SubClassName=ps_output  LeftPortType=input  RightPortType=output  PseudoPeriodic=off  Frequencies=[]  Unit=inherit  AffineConversion=off
  PS-Simulink Converter2 : nesl_utility/PS-Simulink Converter  PhysicalDomain=network_engine_domain  SubClassName=ps_output  LeftPortType=input  RightPortType=output  PseudoPeriodic=off  Frequencies=[]  Unit=inherit  AffineConversion=off
  Pulley-End Alignment1 : Subsystem  AncestorBlock=sm_cable_robot_lib/Pulley-End Alignment  mask(Pulley-End Alignment){majorRadius=0.003, minorRadius=0.001, rho=7800, color=[0.3 0.3 0.3]}
      mask prompts: majorRadius "Ring Major Radius (m)"; minorRadius "Ring Minor Radius (m)"; rho "Ring Density (kg/m^3)"; color "Ring Color [r g b]"
      mask help:
      | This block models the enforced alignment between the belt-cable end attached to the mover and the corresponding column pulley. The block maintains the alignment between the belt-cable and the column pulley such that the belt-cable is always in the x-y plane of the column pulley.
      |
      | Port P corresponds to the pulley reference frame. Port E corresponds to the belt-cable end reference frame.
      mask init:
      | theta = linspace(0, 2 * pi, 20);
      | 
      | crossSection = [minorRadius * cos(theta) + majorRadius;...
      |                 minorRadius * sin(theta)]';
      mask DialogControl Tab1 Prompt: Dimensions
      mask DialogControl Tab2 Prompt: Material Properties
      mask Display: image(fullfile(matlabroot,'toolbox','physmod','sm','smdemos','cable_robot','images','sm_cable_robot_pulley_end_alignment.png'));
  Pulley-End Alignment2 : Subsystem  AncestorBlock=sm_cable_robot_lib/Pulley-End Alignment  mask(Pulley-End Alignment){majorRadius=0.003, minorRadius=0.001, rho=7800, color=[0.3 0.3 0.3]}
      mask prompts: majorRadius "Ring Major Radius (m)"; minorRadius "Ring Minor Radius (m)"; rho "Ring Density (kg/m^3)"; color "Ring Color [r g b]"
      mask help:
      | This block models the enforced alignment between the belt-cable end attached to the mover and the corresponding column pulley. The block maintains the alignment between the belt-cable and the column pulley such that the belt-cable is always in the x-y plane of the column pulley.
      |
      | Port P corresponds to the pulley reference frame. Port E corresponds to the belt-cable end reference frame.
      mask init:
      | theta = linspace(0, 2 * pi, 20);
      | 
      | crossSection = [minorRadius * cos(theta) + majorRadius;...
      |                 minorRadius * sin(theta)]';
      mask DialogControl Tab1 Prompt: Dimensions
      mask DialogControl Tab2 Prompt: Material Properties
      mask Display: image(fullfile(matlabroot,'toolbox','physmod','sm','smdemos','cable_robot','images','sm_cable_robot_pulley_end_alignment.png'));
  Rigid Transform : sm_lib/Frames and Transforms/Rigid Transform  TranslationMethod=StandardAxis  TranslationStandardOffset=0.03535  TranslationLengthUnit=m  TranslationStandardAxis=+Z  TranslationCartesianOffset=[0 0 0]  TranslationROffset=0  TranslationROffsetUnits=m  TranslationZOffset=0  TranslationZOffsetUnits=m  TranslationThetaOffset=0  TranslationThetaOffsetUnits=deg  RotationMethod=None  RotationAngleUnits=deg  RotationStandardAxis=+Z  RotationAngle=0.0  RotationArbitraryAxis=[0 0 1]  FollAlignAxisA=+X  BaseAlignAxisA=+Y  FollAlignAxisB=+Y  BaseAlignAxisB=+Z  RotationSequenceAxes=FollowerAxes  RotationSequence=XYX  RotationSequenceAngles=[0 0 0]  RotationSequenceAnglesUnits=deg  RotationMatrix=[1 0 0; 0 1 0; 0 0 1]
  Rigid Transform1 : sm_lib/Frames and Transforms/Rigid Transform  TranslationMethod=StandardAxis  TranslationStandardOffset=0.03535  TranslationLengthUnit=m  TranslationStandardAxis=-Z  TranslationCartesianOffset=[0 0 0]  TranslationROffset=0  TranslationROffsetUnits=m  TranslationZOffset=0  TranslationZOffsetUnits=m  TranslationThetaOffset=0  TranslationThetaOffsetUnits=deg  RotationMethod=None  RotationAngleUnits=deg  RotationStandardAxis=+Z  RotationAngle=0.0  RotationArbitraryAxis=[0 0 1]  FollAlignAxisA=+X  BaseAlignAxisA=+Y  FollAlignAxisB=+Y  BaseAlignAxisB=+Z  RotationSequenceAxes=FollowerAxes  RotationSequence=XYX  RotationSequenceAngles=[0 0 0]  RotationSequenceAnglesUnits=deg  RotationMatrix=[1 0 0; 0 1 0; 0 0 1]
  Spring and Damper Force1 : sm_lib/Forces and Torques/Spring and Damper Force  NaturalLength=2  NaturalLengthUnits=m  SpringStiffness=115  SpringStiffnessUnits=N/m  DampingCoefficient=0.2  DampingCoefficientUnits=N/(m/s)  SenseForce=on
  Spring and Damper Force2 : sm_lib/Forces and Torques/Spring and Damper Force  NaturalLength=2  NaturalLengthUnits=m  SpringStiffness=150  SpringStiffnessUnits=N/m  DampingCoefficient=0.2  DampingCoefficientUnits=N/(m/s)  SenseForce=on
  Upper Cable End : sm_lib/Belts and Cables/Belt-Cable End
      settings: SourceProductBaseCode=MS
  Upper Cable Properties : sm_lib/Belts and Cables/Belt-Cable Properties  DrumBeltCableAlignment=MonitoredPlanar  GraphicType=PitchLine  GraphicVisPropType=SimpleVisualProperties  GraphicDiffuseColor=[1.0 1.0 1.0]  GraphicSpecularColor=[0.5 0.5 0.5 1.0]  GraphicAmbientColor=[0.15 0.15 0.15 1.0]  GraphicEmissiveColor=[0.0 0.0 0.0 1.0]  GraphicShininess=75  GraphicOpacity=1.0
      settings: SourceProductBaseCode=MS
  Upper Motor Spool : sm_lib/Belts and Cables/Belt-Cable Spool  PitchRadius=0.018  PitchRadiusUnits=m  SenseSpoolAngleA=off  SenseFleetAngleA=off
      settings: SourceProductBaseCode=MS
  LE : PMIOPort  Side=Right
  UE : PMIOPort  Port=2  Side=Right
  B1 : PMIOPort  Port=3  Side=Left
  tag scope: f2=global, f6=global
  wires:
  PS-Simulink Converter1/1 -> [f6]
  PS-Simulink Converter2/1 -> [f2]
  connections:
  Rigid Transform1/LConn1 -- Spring and Damper Force2/LConn1 -- Rigid Transform/LConn1 -- Spring and Damper Force1/LConn1 -- Lower Motor Assembly1/RConn1
  Column Upper Pulley/LConn1 -- Spring and Damper Force2/RConn1 -- CUP Alignment/RConn1 -- Pulley-End Alignment1/LConn1
  Upper Cable Properties/LConn1 -- Column Upper Pulley/RConn2 -- Upper Motor Spool/RConn1
  Pulley-End Alignment1/RConn1 -- UE/RConn1 -- Upper Cable End/LConn1
  Column Upper Pulley xForm/LConn1 -- Column/RConn1
  B1/RConn1 -- Base Offset/RConn1
  Upper Cable End/RConn1 -- Column Upper Pulley/RConn1
  Beam/LConn1 -- Beam xForm/RConn1
  Beam xForm/LConn1 -- Column/RConn2
  Base Offset/LConn1 -- Column/LConn2 -- Beam Upper Pulley xForm2/LConn1
  Column Lower Pulley/RConn2 -- Lower Cable End/RConn1
  Lower Cable Properties/LConn1 -- Lower Motor Spool/RConn1 -- Column Lower Pulley/RConn1
  Lower Motor Assembly1/LConn1 -- Beam Upper Pulley xForm2/RConn1
  Rigid Transform1/RConn1 -- Lower Motor Spool/LConn1
  Rigid Transform/RConn1 -- Upper Motor Spool/LConn1
  Pulley-End Alignment2/RConn1 -- Lower Cable End/LConn1 -- LE/RConn1
  Column/LConn1 -- Column Upper Pulley xForm1/LConn1
  Column Upper Pulley and Right-Angle Bracket Assembly/RConn1 -- CUP Alignment/LConn1
  Column Upper Pulley and Right-Angle Bracket Assembly2/LConn1 -- Column Upper Pulley xForm1/RConn1
  Column Lower Pulley/LConn1 -- Spring and Damper Force1/RConn1 -- Column Upper Pulley and Right-Angle Bracket Assembly2/RConn1 -- Pulley-End Alignment2/LConn1
  Column Upper Pulley and Right-Angle Bracket Assembly/LConn1 -- Column Upper Pulley xForm/RConn1
  PS-Simulink Converter1/LConn1 -- Spring and Damper Force1/RConn2
  PS-Simulink Converter2/LConn1 -- Spring and Damper Force2/RConn2
